simulink model "Auto_mode"  (R2017a)
settings: Solver=VariableStepAuto  StartTime=0.0  StopTime=30  FixedStep=Ts  RelTol=1e-3  EnableMultiTasking=on
model workspace (MAT data in the model file):
  MCOS : class17 (value not decoded)
  MCOS : class17 (value not decoded)
  MCOS : class17 (value not decoded)
  MCOS : class17 (value not decoded)
  MCOS : class17 (value not decoded)
  MCOS : class17 (value not decoded)
  MCOS : class17 (value not decoded)
  MCOS : class17 (value not decoded)
  MCOS : class17 (value not decoded)
  MCOS : class17 (value not decoded)
  MCOS : class17 (value not decoded)
  MCOS : class17 (value not decoded)
  MCOS : class17 (value not decoded)
  MCOS : class17 (value not decoded)
  MCOS : class17 (value not decoded)
  MCOS : class17 (value not decoded)
  false = 0
  MCOS : class17 (value not decoded)
  MCOS : class17 (value not decoded)
  MCOS : class17 (value not decoded)
  MCOS : class17 (value not decoded)
  MCOS : class17 (value not decoded)
  MCOS : class17 (value not decoded)
  MCOS : class17 (value not decoded)
  MCOS : class17 (value not decoded)
  MCOS : class17 (value not decoded)
  MCOS : class17 (value not decoded)
  MCOS : class17 (value not decoded)
  MCOS : class17 (value not decoded)
  MCOS : class17 (value not decoded)
  MCOS : class17 (value not decoded)
  MCOS : class17 (value not decoded)
  MCOS : class17 (value not decoded)
  MCOS : class17 (value not decoded)
  MCOS : class17 (value not decoded)
  MCOS : class17 (value not decoded)
  MCOS : class17 (value not decoded)
  MCOS : class17 (value not decoded)
  MCOS : class17 (value not decoded)
  MCOS : class17 (value not decoded)
  MCOS : class17 (value not decoded)
  MCOS : class17 (value not decoded)
  MCOS : class17 (value not decoded)
  MCOS : class17 (value not decoded)
  MCOS : class17 (value not decoded)
  MCOS : class17 (value not decoded)
  MCOS : class17 (value not decoded)
  MCOS : class17 (value not decoded)
  MCOS : class17 (value not decoded)
  MCOS : class17 (value not decoded)
  MCOS : class17 (value not decoded)
  MCOS : class17 (value not decoded)
  MCOS : class17 (value not decoded)
  MCOS : class17 (value not decoded)
  MCOS : class17 (value not decoded)
  MCOS : class17 (value not decoded)
  MCOS : class17 (value not decoded)
  MCOS : class17 (value not decoded)
  MCOS : class17 (value not decoded)
  MCOS : class17 (value not decoded)
  MCOS : class17 (value not decoded)
  MCOS : class17 (value not decoded)
  true = 1
  MCOS : class17 (value not decoded)
  variableType = 'S'
  MCOS : class17 (value not decoded)
  MCOS : class17 (value not decoded)
  MCOS : class17 (value not decoded)
  MCOS : class17 (value not decoded)
  MCOS : class17 (value not decoded)
  MCOS : class17 (value not decoded)
  MCOS : class17 (value not decoded)
  MCOS : class17 (value not decoded)
  MCOS : class17 (value not decoded)
  MCOS : class17 (value not decoded)
  MCOS : class17 (value not decoded)
  MCOS : class17 (value not decoded)
  MCOS : class17 (value not decoded)
  MCOS : class17 (value not decoded)
undefined symbols (not defined in the file or in its folder): Outer_Ts, sensor_max_range, sensor_min_range, Ts
libraries: simulink x8, aerolibactuator x4, vrlib x2, aerolibanim x2, shared6dof x1, aerolibwind2 x1, aerolibnav x1, sharedutil x1, aerolibconvert2 x1, dspbuff3 x1
(part 2 of 2)

== system Auto_mode/Sensor Implementation/west sensor implementation ==
  actual_distance : Inport
  Band-Limited White Noise : simulink/Sources/Band-Limited White Noise  Cov=[0.01]  Ts=0.1  seed=[600]
  Measurement Limits1 : Saturate  UpperLimit=sensor_max_range  LowerLimit=sensor_min_range
  Sum : Sum  Inputs=|++
  noise : Scope
  measured_distance : Outport
  wires:
  actual_distance/1 -> Sum/1  "actual_distance"
  Measurement Limits1/1 -> measured_distance/1  "measured_distance"
  Band-Limited White Noise/1 -> noise/1, Sum/2
  Sum/1 -> Measurement Limits1/1

== matlab function Auto_mode/Thrust Controller/desired_accel_vector_earth_length ==
  data: u input; length output
function length = vectorLength(u)
%#codegen


length = sqrt( ((u(1))^2) + ((u(2))^2) + ((u(3))^2) );

== matlab function Auto_mode/Thrust Controller/Vector Size2 ==
  data: u input; length output
function length = vectorLength(u)
%#codegen


length = sqrt( ((u(1))^2) + ((u(2))^2) + ((u(3))^2) );

== matlab function Auto_mode/Gravity and Drag Distrubance Calculation ==
  data: DCMeb input; FGx output; Vb input; FGy output; FGz output; FDx output; FDy output; FDz output
function [FGx, FGy, FGz, FDx, FDy, FDz] = gravityDragCalculation(DCMeb, Vb)
%   Gravity and Drag Calculations
%   Inputs
%   DCMbe = Direct Cosine Matrix, from earth to body
%   Vb = Linear Velocity, body frame
%   Outputs
%   FGa = Force of gravity in the 'a' axis, body frame
%   FDa = Force of drag in the 'a' axis, body frame

%% Gravity
%Gravity Constants
mass = 3.352;
gravityForce_earth = [0, 0, (9.81*mass)];

%Gravity Calculations
FG = DCMeb*transpose(gravityForce_earth);
FGx = FG(1);
FGy = FG(2);
FGz = FG(3);

%% Drag
%Drag Constants
airDensity          = 1.1644;                                               %wikipedia air density at 30 degrees C
dragCoefficient     = 1.0;                                                  %SLADe
surfaceArea         = [0.1 0.5 0.7];                                        %Drone 3 measurements
Vbx = Vb(1);
Vby = Vb(2);                                                               
Vbz = Vb(3);

Vbxdir = 0;
Vbydir = 0;
Vbzdir = 0;

if Vb(1) ~= 0
    Vbxdir = (Vb(1)/abs(Vb(1)));
end
if Vb(2) ~= 0
    Vbydir = (Vb(2)/abs(Vb(2)));
end
if Vb(3) ~= 0
    Vbzdir = (Vb(3)/abs(Vb(3)));
end


%Drag Calculations
FDx = 0.5 * airDensity * (Vbx^2) * dragCoefficient * surfaceArea(1) * -Vbxdir;
FDy = 0.5 * airDensity * (Vby^2) * dragCoefficient * surfaceArea(2) * -Vbydir;
FDz = 0.5 * airDensity * (Vbz^2) * dragCoefficient * surfaceArea(3) * -Vbzdir;

== matlab function Auto_mode/Thrust Controller/current_accel_vector_body_length ==
  data: u input; length output
function length = vectorLength(u)
%#codegen


length = sqrt( ((u(1))^2) + ((u(2))^2) + ((u(3))^2) );

== matlab function Auto_mode/Motor Mixer ==
  data: Z input; phi input; theta input; T1 output; T2 output; psi input; T3 output; T4 output
function [T1,T2,T3,T4]  = MotorMixer(Z, phi, theta, psi)
%       ccw       cw            
%N         3    1
%           \  /
%            \/
%            /\
%           /  \
%          2    4       
%       cw        ccw   E
%%%%%%%%%%%%%%%%%%%%%%%%%

%% Inputs
armLength           = 0.41;            %Meters
alpha               = deg2rad(15);     %Rad
chordLength         = 0.040;           %Meters
liftDragRatio       = 0.1;

roll_arm    = armLength * sin(alpha);
pitch_arm   = armLength * cos(alpha);
yaw_arm     = chordLength/liftDragRatio;
%% 

roll_contribution   = [-roll_arm roll_arm roll_arm -roll_arm];
pitch_contribution  = [pitch_arm -pitch_arm pitch_arm -pitch_arm];
yaw_contribution    = [-yaw_arm -yaw_arm yaw_arm yaw_arm];

contribution_matrix = [1 1 1 1; roll_contribution; pitch_contribution; yaw_contribution];

thrust_matrix = inv(contribution_matrix)*[Z;phi;theta;psi];

T1 = thrust_matrix(1,1);
T2 = thrust_matrix(2,1);
T3 = thrust_matrix(3,1);
T4 = thrust_matrix(4,1);

== matlab function Auto_mode/Motor Thrust Calculation ==
  data: T1 input; Z output; T2 input; T3 input; T4 input; L output; M output; N output
function [Z, L, M, N]  = MotorThrustCalculation(T1,T2,T3,T4)
%       ccw       cw            
%N         3    1
%           \  /
%            \/
%            /\
%           /  \
%          2    4       
%       cw        ccw   E
%%%%%%%%%%%%%%%%%%%%%%%%%

%% Inputs
armLength           = 0.41;            %Meters
alpha               = deg2rad(15);     %Rad
chordLength         = 0.040;           %Meters
liftDragRatio       = 0.1;

roll_arm    = armLength * sin(alpha);
pitch_arm   = armLength * cos(alpha);
yaw_arm     = chordLength/liftDragRatio;
%% 

roll_contribution   = [-roll_arm roll_arm roll_arm -roll_arm];
pitch_contribution  = [pitch_arm -pitch_arm pitch_arm -pitch_arm];
yaw_contribution    = [-yaw_arm -yaw_arm yaw_arm yaw_arm];

contribution_matrix = [1 1 1 1; roll_contribution; pitch_contribution; yaw_contribution];

moment_matrix = (contribution_matrix)*[T1;T2;T3;T4];

Z = moment_matrix(1,1);
L = moment_matrix(2,1);
M = moment_matrix(3,1);
N = moment_matrix(4,1);

== matlab function Auto_mode/Waypoint Generator NED/pos_check ==
  data: current_wp input; current_pos input; pop_next_wp output; count input; count output; current_count output
function [pop_next_wp, count, current_count] = pos_check(current_wp, current_pos, count)

reached_waypoint_threshold = 0.5;                                             %metres, distance that confirms, wp has been reached
count_threshold = 1;

pop_next_wp = 0;

current_count = 0;

for i=1:3
    if abs(current_pos(i) - current_wp(i)) <= reached_waypoint_threshold              %If we have reached the threshold, trigger rising edge. I.e send out next waypoint
        current_count = current_count + 1;
        %pop_next_wp = 1;
    else
    end
end

if current_count == 3
    count = count + 1;
else
    count = 0;
end

if count > count_threshold
    pop_next_wp = 1;
    count = 0;
end

== matlab function Auto_mode/Near Wall Disturbance ==
  data: earth_linear_position_absolute input; dcm input; T1 input; Tnw1 output; T2 input; T3 input; T4 input; Tnw2 output; Tnw3 output; Tnw4 output
function [Tnw1, Tnw2, Tnw3, Tnw4]  = nearWall(earth_linear_position_absolute, dcm, T1, T2, T3, T4)

%% Place the Rotors
%  Use absolute position. Offset rotors by arm length and dcm. 
%       ccw       cw            
%N         3    1
%           \  /
%            \/
%            /\
%           /  \
%          2    4       
%       cw        ccw   E
%%%%%%%%%%%%%%%%%%%%%%%%%

%% Inputs
armLength           = 0.41;            %Meters
alpha               = deg2rad(15);     %Rad

roll_arm    = armLength * sin(alpha);
pitch_arm   = armLength * cos(alpha);


%%  First assume no rotation to simplify
%  rotor_pos = [Npos ±Noffset; Epos ±Eoffset; Dpos]
rotor_pos = zeros([4 3]);
rotor_pos(1, 1:3) = [earth_linear_position_absolute(1)+pitch_arm earth_linear_position_absolute(2)+roll_arm earth_linear_position_absolute(3)];
rotor_pos(2, 1:3) = [earth_linear_position_absolute(1)-pitch_arm earth_linear_position_absolute(2)-roll_arm earth_linear_position_absolute(3)];
rotor_pos(3, 1:3) = [earth_linear_position_absolute(1)+pitch_arm earth_linear_position_absolute(2)-roll_arm earth_linear_position_absolute(3)];
rotor_pos(4, 1:3) = [earth_linear_position_absolute(1)-pitch_arm earth_linear_position_absolute(2)+roll_arm earth_linear_position_absolute(3)];

rotor_distance_from_north_wall = zeros([4 1]);
rotor_distance_from_south_wall = zeros([4 1]);
rotor_distance_from_east_wall = zeros([4 1]);
rotor_distance_from_west_wall = zeros([4 1]);
closest_wall = zeros([4 1]);
disturbance_percentage = zeros([4 1]);

%% North wall
if earth_linear_position_absolute(2) <= -2
    north_wall = 8;
elseif earth_linear_position_absolute(2) > -2
    north_wall = earth_linear_position_absolute(2) + 10;              %y = x + 10 start sloping at N = 8, E = 2
else
    north_wall = 8;
end

%% South Wall 
if earth_linear_position_absolute(2) <= 2
    south_wall = -1;
elseif earth_linear_position_absolute(2) > 2
    south_wall = earth_linear_position_absolute(2) + 6;              %y = x + 10 start sloping at N = 8, E = -2
else
    south_wall = -1;
end
    
%% West Wall 
if earth_linear_position_absolute(1) <= 8
    west_wall = -2;
elseif earth_linear_position_absolute(1) > 8
    west_wall = earth_linear_position_absolute(1) - 10;              %y = x + 10 start sloping at N = 8, E = -2
else
    west_wall = -2;
end

%% East Wall 
if earth_linear_position_absolute(1) <= 2
    east_wall = 2;
elseif earth_linear_position_absolute(1) > 2
    east_wall = earth_linear_position_absolute(1) - 6;              %y = x + 10 start sloping at N = 8, E = -2
else
    east_wall = 2;
end

for i = 1:4
    rotor_distance_from_north_wall(i)   = abs(north_wall - rotor_pos(i, 1));
    rotor_distance_from_south_wall(i)   = abs(south_wall - rotor_pos(i, 1));
    rotor_distance_from_east_wall(i)    = abs(east_wall - rotor_pos(i, 2));
    rotor_distance_from_west_wall(i)    = abs(west_wall - rotor_pos(i, 2));
    
    closest_wall(i) = min([rotor_distance_from_north_wall(i) rotor_distance_from_south_wall(i) rotor_distance_from_east_wall(i) rotor_distance_from_west_wall(i)]);
    
    if closest_wall(i) <= 1
        disturbance_percentage(i) = 0.1 - closest_wall(i)*0.1;
    else
        disturbance_percentage(i) = 0;
    end
end


Tnw1 = T1 * disturbance_percentage(1);
Tnw2 = T2 * disturbance_percentage(2);
Tnw3 = T3 * disturbance_percentage(3);
Tnw4 = T4 * disturbance_percentage(4);

== matlab function Auto_mode/Sensor Implementation/Proximity ==
  data: n input; s input; pv output; e input; w input; f input; r input
function pv = proximityVector(n, s, e, w, f, r)


x = n-s;
y = e-w;
z = f-r;

pv = [x y z];

== matlab function Auto_mode/Sensor Implementation/North Wall Function ==
  data: ypos input; north_wall output
function north_wall = NW(ypos)

if ypos <= -2
    north_wall = 8;
elseif ypos > -2
    north_wall = ypos + 10;              %y = x + 10 start sloping at N = 8, E = 2
else
    north_wall = 8;
end

== matlab function Auto_mode/Sensor Implementation/South Wall Function ==
  data: ypos input; south_wall output
function south_wall = NW(ypos)


if ypos <= 2
    south_wall = -1;
elseif ypos > 2
    south_wall = ypos + 6;              %y = x + 10 start sloping at N = 8, E = 2
else
    south_wall = -1;
end

== matlab function Auto_mode/Sensor Implementation/East Wall Function ==
  data: xpos input; east_wall output
function east_wall = NW(xpos)


if xpos <= 8
    east_wall = 2;
elseif xpos > 8
    east_wall = xpos - 6;              %y = x + 10 start sloping at N = 8, E = 2
else
    east_wall = 2;
end

== matlab function Auto_mode/Sensor Implementation/West Wall Function ==
  data: xpos input; west_wall output
function west_wall = NW(xpos)


if xpos <= 8
    west_wall = -2;
elseif xpos > 8
    west_wall = xpos - 10;              %y = x + 10 start sloping at N = 8, E = -2
else
    west_wall = -2;
end
